simulink model "SegheriaSCADA2"  (R2024b)
settings: Solver=FixedStepAuto  StartTime=0.0  StopTime=2000  FixedStep=0.025  RelTol=1e-3
values from neighbouring files (symbols this model uses):
  b = t + 2*s    (= 3.6)    [ParametriSegheria.m]    (also in ParametriSegheriaDinamica.m; main_param_CLASSIC.m; main_param_SCADA.m)
  b2 = t2 + 2*s2    (= 10)    [ParametriSegheria.m]    (also in ParametriSegheriaDinamica.m; main_param_CLASSIC.m; main_param_SCADA.m)
  h_index = [70, 80, 90, 100]    [ParametriSegheria.m]    (also in ParametriSegheriaDinamica.m = [80, 90, 100]; main_param_CLASSIC.m = [80, 90, 100, 110]; main_param_SCADA.m = [80, 90, 100, 110])
  h_start_1 = 1    [main_param_CLASSIC.m]
  h_start_2 = 2    [main_param_CLASSIC.m]
  h_start_3 = 3    [main_param_CLASSIC.m]
  h_start_4 = 1    [main_param_CLASSIC.m]
  h_start_5 = 2    [main_param_CLASSIC.m]
  h_start_6 = 3    [main_param_CLASSIC.m]
  i_id = 60    [ParametriSegheria.m]
  i_id2 = 60    [ParametriSegheria.m]
  i_max = 100    [ParametriSegheria.m]
  kc = [0 35 40 50 55 90]    [ParametriSegheria.m]    (also in ParametriSegheriaDinamica.m = [0, 25, 30, 35, 50, 70]; main_param_CLASSIC.m = [0, 25, 30, 35, 50, 70]; main_param_SCADA.m = [0, 25, 30, 35, 50, 70])
  Kt = 2    [ParametriSegheria.m]    (also in ParametriSegheriaDinamica.m = 10000; main_param_CLASSIC.m = 10000; main_param_SCADA.m = 10000)
  Kt2 = 5    [ParametriSegheria.m]    (also in ParametriSegheriaDinamica.m = 4500; main_param_CLASSIC.m = 4500; main_param_SCADA.m = 4500)
  l_index = [20, 30, 40, 50]    [ParametriSegheria.m]    (also in ParametriSegheriaDinamica.m = [30, 40, 50]; main_param_CLASSIC.m = [30, 40, 50, 60]; main_param_SCADA.m = [30, 40, 50, 60])
  l_start_1 = 1    [main_param_CLASSIC.m]
  l_start_2 = 1    [main_param_CLASSIC.m]
  l_start_3 = 1    [main_param_CLASSIC.m]
  l_start_4 = 1    [main_param_CLASSIC.m]
  l_start_5 = 1    [main_param_CLASSIC.m]
  l_start_6 = 1    [main_param_CLASSIC.m]
  Lt = 4    [ParametriSegheria.m]    (also in ParametriSegheriaDinamica.m; main_param_CLASSIC.m; main_param_SCADA.m)
  Mag_D1 = [0 randi([220 500], 1, 40)]    [ParametriSegheria.m]    (also in ParametriSegheriaDinamica.m = [0 randi([200 500], 1, N_log)]; main_param_CLASSIC.m = [0 randi([200 500], 1, N_log)]; main_param_SCADA.m = [0 randi([200 500], 1, N_log)])
  Mag_D2 = [0 randi([220 500], 1, 40)]    [ParametriSegheria.m]    (also in ParametriSegheriaDinamica.m = [0 randi([200 500], 1, N_log)]; main_param_CLASSIC.m = [0 randi([200 500], 1, N_log)]; main_param_SCADA.m = [0 randi([200 500], 1, N_log)])
  Mag_D3 = [0 randi([220 500], 1, 40)]    [ParametriSegheria.m]    (also in ParametriSegheriaDinamica.m = [0 randi([200 500], 1, N_log)]; main_param_CLASSIC.m = [0 randi([200 500], 1, N_log)]; main_param_SCADA.m = [0 randi([200 500], 1, N_log)])
  Mag_legno1 = [0 randi([1 5], 1, 40)]    [ParametriSegheria.m]    (also in ParametriSegheriaDinamica.m = [0 randi([1 5], 1, N_log)]; main_param_CLASSIC.m = [0 randi([1 5], 1, N_log)]; main_param_SCADA.m = [0 randi([1 5], 1, N_log)])
  Mag_legno2 = [0 randi([1 5], 1, 40)]    [ParametriSegheria.m]    (also in ParametriSegheriaDinamica.m = [0 randi([1 5], 1, N_log)]; main_param_CLASSIC.m = [0 randi([1 5], 1, N_log)]; main_param_SCADA.m = [0 randi([1 5], 1, N_log)])
  Mag_legno3 = [0 randi([1 5], 1, 40)]    [ParametriSegheria.m]    (also in ParametriSegheriaDinamica.m = [0 randi([1 5], 1, N_log)]; main_param_CLASSIC.m = [0 randi([1 5], 1, N_log)]; main_param_SCADA.m = [0 randi([1 5], 1, N_log)])
  n_sottili = 4    [ParametriSegheria.m]
  omega = 50    [ParametriSegheria.m]
  omega2 = 3000*(2*pi/60)    (= 314.159265359)    [ParametriSegheria.m]
  SR = Rs/Rm    (= 5.33333333333)    [ParametriSegheria.m]    (also in ParametriSegheriaDinamica.m; main_param_CLASSIC.m; main_param_SCADA.m)
  SR2 = Rc/Rm2    (= 4)    [ParametriSegheria.m]    (also in ParametriSegheriaDinamica.m; main_param_CLASSIC.m; main_param_SCADA.m)
  thrsh = 40    [ParametriSegheria.m]
  Tloss = Tatt+ Tdamp    (= 17.3333333333)    [ParametriSegheria.m]
  Tloss2 = Tatt2+ Tdamp2    (= 66.8318530718)    [ParametriSegheria.m]
libraries: simulink x15, slpidlib x9
(part 2 of 3)

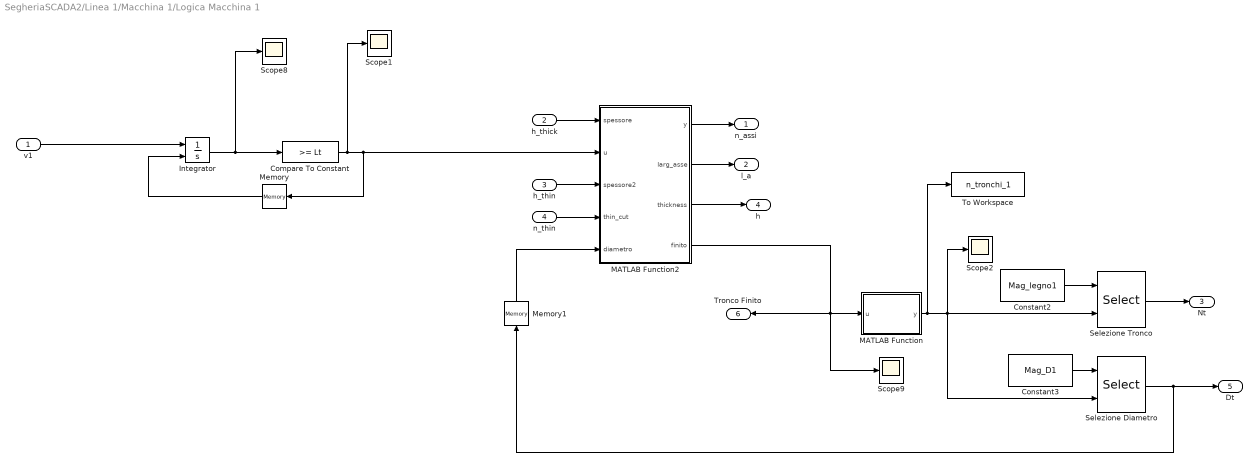
== system SegheriaSCADA2/Linea 1/Macchina 1/Logica Macchina 1 ==
  v1 : Inport
  h_thick : Inport  Port=2
  h_thin : Inport  Port=3
  n_thin : Inport  Port=4
  Compare To Constant : simulink/Logic and Bit Operations/Compare To Constant  relop=>=  const=Lt  OutDataTypeStr=boolean
  Constant2 : Constant  Value=Mag_legno1
  Constant3 : Constant  Value=Mag_D1
  Integrator : Integrator  ExternalReset=rising
  MATLAB Function : MATLAB Function  TreatAsAtomicUnit=on
  MATLAB Function2 : MATLAB Function  TreatAsAtomicUnit=on
  Memory : Memory
  Memory1 : Memory
  Scope{1..2,8..9} (4 alike) : Scope
  Selezione Diametro : Selector  IndexMode=Zero-based  InputPortWidth=length(Mag_D1)  IndexOptions=Index vector (port)  Indices=[1 3]  OutputSizes=1
  Selezione Tronco : Selector  IndexMode=Zero-based  InputPortWidth=length(Mag_legno1)  IndexOptions=Index vector (port)  Indices=[1 3]  OutputSizes=1
  To Workspace : ToWorkspace  VariableName=n_tronchi_1  SaveFormat=Timeseries  SampleTime=-1
  n_assi : Outport
  l_a : Outport  Port=2
  Nt : Outport  Port=3
  h : Outport  Port=4
  Dt : Outport  Port=5
  Tronco Finito : Outport  Port=6
  wires:
  Selezione Diametro/1 -> Dt/1, Memory1/1
  MATLAB Function2/4(finito) -> Scope9/1, Tronco Finito/1, MATLAB Function/1(u)
  Memory/1 -> Integrator/2
  Memory1/1 -> MATLAB Function2/5(diametro)
  Constant2/1 -> Selezione Tronco/1
  v1/1 -> Integrator/1
  Integrator/1 -> Compare To Constant/1, Scope8/1
  Constant3/1 -> Selezione Diametro/1
  MATLAB Function/1(y) -> To Workspace/1, Selezione Diametro/2, Scope2/1, Selezione Tronco/2
  MATLAB Function2/1(y) -> n_assi/1
  Selezione Tronco/1 -> Nt/1
  MATLAB Function2/2(larg_asse) -> l_a/1
  Compare To Constant/1 -> Scope1/1, Memory/1, MATLAB Function2/2(u)
  h_thick/1 -> MATLAB Function2/1(spessore)
  h_thin/1 -> MATLAB Function2/3(spessore2)
  n_thin/1 -> MATLAB Function2/4(thin_cut)
  MATLAB Function2/3(thickness) -> h/1

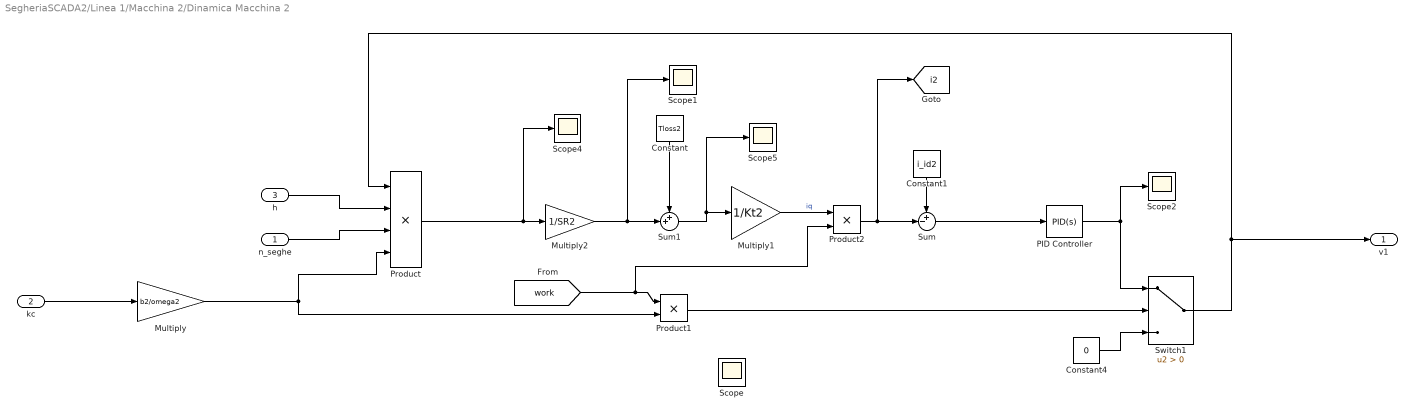
== system SegheriaSCADA2/Linea 1/Macchina 2/Dinamica Macchina 2 ==
  n_seghe : Inport
  kc : Inport  Port=2
  h : Inport  Port=3
  Constant : Constant  Value=Tloss2
  Constant1 : Constant  Value=i_id2
  Constant4 : Constant  Value=0
  Multiply : Gain  Gain=b2/omega2
  Multiply1 : Gain  Gain=1/Kt2
  Multiply2 : Gain  Gain=1/SR2
  PID Controller : slpidlib/PID Controller  Controller=PID  Form=Parallel  TimeDomain=Continuous-time  UseExternalTs=off  SampleTime=-1  IntegratorMethod=Forward Euler  FilterMethod=Forward Euler  ControllerParametersSource=internal  P=0.1  I=0  UseKiTs=off  D=0  UseExternalDerivativeSource=off  N=100  UseFilter=on  TunerSelectOption=Transfer Function Based (PID Tuner App)  InitialConditionSource=internal  InitialConditionForIntegrator=0  InitialConditionForFilter=0  DifferentiatorICPrevScaledInput=0  ExternalReset=none  TrackingMode=off  Kt=1  LimitOutput=off  SatLimitsSource=internal  UpperSaturationLimit=1.7  LowerSaturationLimit=0  LinearizeAsGain=on  AntiWindupMode=none  Kb=1  LimitIntegrator=off  UpperIntegratorSaturationLimit=inf  LowerIntegratorSaturationLimit=-inf  POutMin=[]  POutMax=[]  IOutMin=[]  IOutMax=[]  DOutMin=[]  DOutMax=[]  NOutMin=[]  NOutMax=[]  SumOutMin=[]  SumOutMax=[]  SaturationOutMin=[]  SaturationOutMax=[]  PParamMin=[]  PParamMax=[]  IParamMin=[]  IParamMax=[]  DParamMin=[]  DParamMax=[]  NParamMin=[]  NParamMax=[]  KbParamMin=[]  KbParamMax=[]  KtParamMin=[]  KtParamMax=[]  KbOutMin=[]  KbOutMax=[]  KtOutMin=[]  KtOutMax=[]  IntegratorOutMin=[]  IntegratorOutMax=[]  FilterOutMin=[]  FilterOutMax=[]  SumI1OutMin=[]  SumI1OutMax=[]  SumI2OutMin=[]  SumI2OutMax=[]  SumI3OutMin=[]  SumI3OutMax=[]  SumI4OutMin=[]  SumI4OutMax=[]  SumDOutMin=[]  SumDOutMax=[]  DifferentiatorOutMin=[]  DifferentiatorOutMax=[]  FilterDiffOutCoefMin=[]  FilterDiffOutCoefMax=[]  ReciprocalOutMin=[]  ReciprocalOutMax=[]  SumDenOutMin=[]  SumDenOutMax=[]  SumNumOutMin=[]  SumNumOutMax=[]  DivideOutMin=[]  DivideOutMax=[]  UdiffTsProdOutMin=[]  UdiffTsProdOutMax=[]  NTsProdOutMin=[]  NTsProdOutMax=[]  UintegralTsProdOutMin=[]  UintegralTsProdOutMax=[]  UngainTsProdOutMin=[]  UngainTsProdOutMax=[]  ClampingZeroOutDataTypeStr=Inherit: Inherit via back propagation  ClampingZeroOutMin=[]  ClampingZeroOutMax=[]  FilterDenConstantOutDataTypeStr=Inherit: Inherit via back propagation  FilterDenConstantOutMin=[]  FilterDenConstantOutMax=[]  PCopyOutDataTypeStr=Inherit: Inherit via back propagation  PCopyOutMin=[]  PCopyOutMax=[]  NCopyOutDataTypeStr=Inherit: Inherit via back propagation  NCopyOutMin=[]  NCopyOutMax=[]  IntegratorContinuousStateAttributes=''  IntegratorStateMustResolveToSignalObject=off  IntegratorRTWStateStorageClass=Auto  FilterContinuousStateAttributes=''  FilterStateMustResolveToSignalObject=off  FilterRTWStateStorageClass=Auto  ParallelPVariant=InternalParameters  IdealPVariant=Disabled  IVariant=InternalParameters  DVariant=InternalParameters  IntegratorVariant=Continuous  SatVariant=Disabled  AWVariant=Passthrough  PCopyVariant=Disabled  TRVariant=Disabled  FdbkBlocksVariant=Forward  IdealPFdbkVariant=Disabled  SatFdbkVariant=Disabled  DerivativeFilterVariant=ContFilter  NVariant=InternalParameters  NCopyVariant=Disabled  FilterICVariant=InternalICsFilter  IntegratorICVariant=InternalICs  ExternalResetVariant=Disabled  TRSumVariant=Passthrough  SumFdbkVariant=Disabled  SumVariant=Sum_PID  TsampFilterVariant=InternalTs  TsampNgainVariant=Passthrough  TsampIntegralVariant=Disabled_SignalSpec  ExternalSaturationOutDataTypeStr=Inherit: Same as second input  DerivativeSourceVariant=ErrorSignal  PreIntVariant=InternalPreInt
  Product : Product  Inputs=4
  Product1 : Product
  Product2 : Product
  Scope{,1..2,4..5} (5 alike) : Scope
  Sum : Sum  Inputs=+-|
  Sum1 : Sum  Inputs=++|
  Switch1 : Switch  Criteria=u2 > Threshold  SaturateOnIntegerOverflow=off  InputSameDT=off
  v1 : Outport
  tag scope: i2=global
  wires:
  Constant4/1 -> Switch1/3
  Product/1 -> Scope4/1, Multiply2/1
  PID Controller/1 -> Switch1/1, Scope2/1
  Multiply1/1 -> Product2/1  "iq"
  kc/1 -> Multiply/1
  Switch1/1 -> v1/1, Product/1
  Constant1/1 -> Sum/1
  Sum/1 -> PID Controller/1
  Multiply2/1 -> Scope1/1, Sum1/2
  Sum1/1 -> Scope5/1, Multiply1/1
  Constant/1 -> Sum1/1
  h/1 -> Product/2
  n_seghe/1 -> Product/3
  Multiply/1 -> Product1/2, Product/4
  Product1/1 -> Switch1/2
  [work] -> Product2/2, Product1/1
  Product2/1 -> [i2], Sum/2

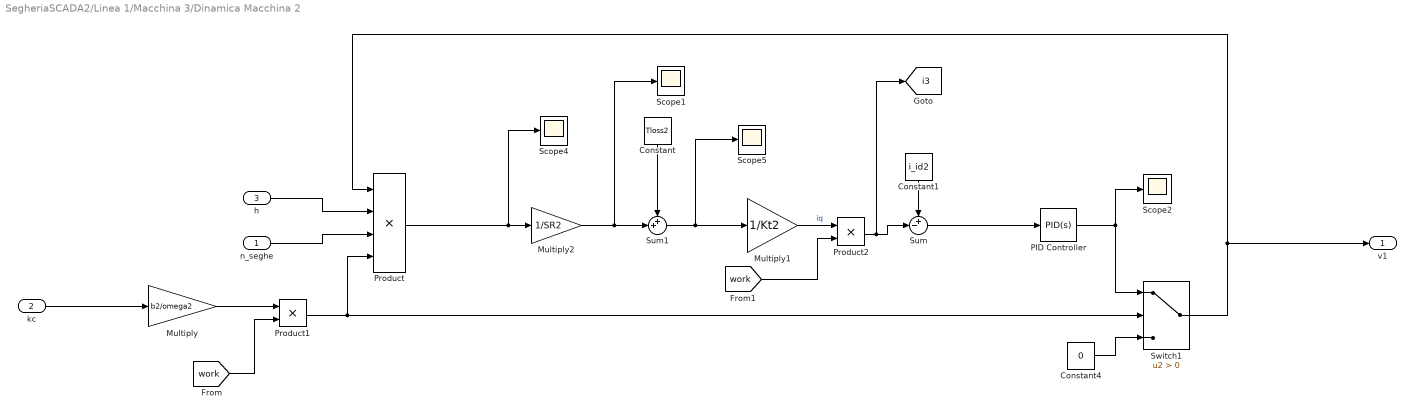
== system SegheriaSCADA2/Linea 1/Macchina 3/Dinamica Macchina 2 ==
  n_seghe : Inport
  kc : Inport  Port=2
  h : Inport  Port=3
  Constant : Constant  Value=Tloss2
  Constant1 : Constant  Value=i_id2
  Constant4 : Constant  Value=0
  Multiply : Gain  Gain=b2/omega2
  Multiply1 : Gain  Gain=1/Kt2
  Multiply2 : Gain  Gain=1/SR2
  PID Controller : slpidlib/PID Controller  Controller=PID  Form=Parallel  TimeDomain=Continuous-time  UseExternalTs=off  SampleTime=-1  IntegratorMethod=Forward Euler  FilterMethod=Forward Euler  ControllerParametersSource=internal  P=0.1  I=0  UseKiTs=off  D=0  UseExternalDerivativeSource=off  N=100  UseFilter=on  TunerSelectOption=Transfer Function Based (PID Tuner App)  InitialConditionSource=internal  InitialConditionForIntegrator=0  InitialConditionForFilter=0  DifferentiatorICPrevScaledInput=0  ExternalReset=none  TrackingMode=off  Kt=1  LimitOutput=off  SatLimitsSource=internal  UpperSaturationLimit=1.7  LowerSaturationLimit=0  LinearizeAsGain=on  AntiWindupMode=none  Kb=1  LimitIntegrator=off  UpperIntegratorSaturationLimit=inf  LowerIntegratorSaturationLimit=-inf  POutMin=[]  POutMax=[]  IOutMin=[]  IOutMax=[]  DOutMin=[]  DOutMax=[]  NOutMin=[]  NOutMax=[]  SumOutMin=[]  SumOutMax=[]  SaturationOutMin=[]  SaturationOutMax=[]  PParamMin=[]  PParamMax=[]  IParamMin=[]  IParamMax=[]  DParamMin=[]  DParamMax=[]  NParamMin=[]  NParamMax=[]  KbParamMin=[]  KbParamMax=[]  KtParamMin=[]  KtParamMax=[]  KbOutMin=[]  KbOutMax=[]  KtOutMin=[]  KtOutMax=[]  IntegratorOutMin=[]  IntegratorOutMax=[]  FilterOutMin=[]  FilterOutMax=[]  SumI1OutMin=[]  SumI1OutMax=[]  SumI2OutMin=[]  SumI2OutMax=[]  SumI3OutMin=[]  SumI3OutMax=[]  SumI4OutMin=[]  SumI4OutMax=[]  SumDOutMin=[]  SumDOutMax=[]  DifferentiatorOutMin=[]  DifferentiatorOutMax=[]  FilterDiffOutCoefMin=[]  FilterDiffOutCoefMax=[]  ReciprocalOutMin=[]  ReciprocalOutMax=[]  SumDenOutMin=[]  SumDenOutMax=[]  SumNumOutMin=[]  SumNumOutMax=[]  DivideOutMin=[]  DivideOutMax=[]  UdiffTsProdOutMin=[]  UdiffTsProdOutMax=[]  NTsProdOutMin=[]  NTsProdOutMax=[]  UintegralTsProdOutMin=[]  UintegralTsProdOutMax=[]  UngainTsProdOutMin=[]  UngainTsProdOutMax=[]  ClampingZeroOutDataTypeStr=Inherit: Inherit via back propagation  ClampingZeroOutMin=[]  ClampingZeroOutMax=[]  FilterDenConstantOutDataTypeStr=Inherit: Inherit via back propagation  FilterDenConstantOutMin=[]  FilterDenConstantOutMax=[]  PCopyOutDataTypeStr=Inherit: Inherit via back propagation  PCopyOutMin=[]  PCopyOutMax=[]  NCopyOutDataTypeStr=Inherit: Inherit via back propagation  NCopyOutMin=[]  NCopyOutMax=[]  IntegratorContinuousStateAttributes=''  IntegratorStateMustResolveToSignalObject=off  IntegratorRTWStateStorageClass=Auto  FilterContinuousStateAttributes=''  FilterStateMustResolveToSignalObject=off  FilterRTWStateStorageClass=Auto  ParallelPVariant=InternalParameters  IdealPVariant=Disabled  IVariant=InternalParameters  DVariant=InternalParameters  IntegratorVariant=Continuous  SatVariant=Disabled  AWVariant=Passthrough  PCopyVariant=Disabled  TRVariant=Disabled  FdbkBlocksVariant=Forward  IdealPFdbkVariant=Disabled  SatFdbkVariant=Disabled  DerivativeFilterVariant=ContFilter  NVariant=InternalParameters  NCopyVariant=Disabled  FilterICVariant=InternalICsFilter  IntegratorICVariant=InternalICs  ExternalResetVariant=Disabled  TRSumVariant=Passthrough  SumFdbkVariant=Disabled  SumVariant=Sum_PID  TsampFilterVariant=InternalTs  TsampNgainVariant=Passthrough  TsampIntegralVariant=Disabled_SignalSpec  ExternalSaturationOutDataTypeStr=Inherit: Same as second input  DerivativeSourceVariant=ErrorSignal  PreIntVariant=InternalPreInt
  Product : Product  Inputs=4
  Product1 : Product
  Product2 : Product
  Scope{1..2,4..5} (4 alike) : Scope
  Sum : Sum  Inputs=+-|
  Sum1 : Sum  Inputs=++|
  Switch1 : Switch  Criteria=u2 > Threshold  SaturateOnIntegerOverflow=off  InputSameDT=off
  v1 : Outport
  tag scope: i3=global
  wires:
  n_seghe/1 -> Product/3
  h/1 -> Product/2
  Constant/1 -> Sum1/1
  Sum1/1 -> Multiply1/1, Scope5/1
  Multiply2/1 -> Sum1/2, Scope1/1
  Sum/1 -> PID Controller/1
  Constant1/1 -> Sum/1
  Switch1/1 -> Product/1, v1/1
  kc/1 -> Multiply/1
  Multiply1/1 -> Product2/1  "iq"
  PID Controller/1 -> Scope2/1, Switch1/1
  Product/1 -> Multiply2/1, Scope4/1
  Constant4/1 -> Switch1/3
  Multiply/1 -> Product1/1
  Product1/1 -> Switch1/2, Product/4
  [work] -> Product1/2
  Product2/1 -> [i3], Sum/2
  [work] -> Product2/2

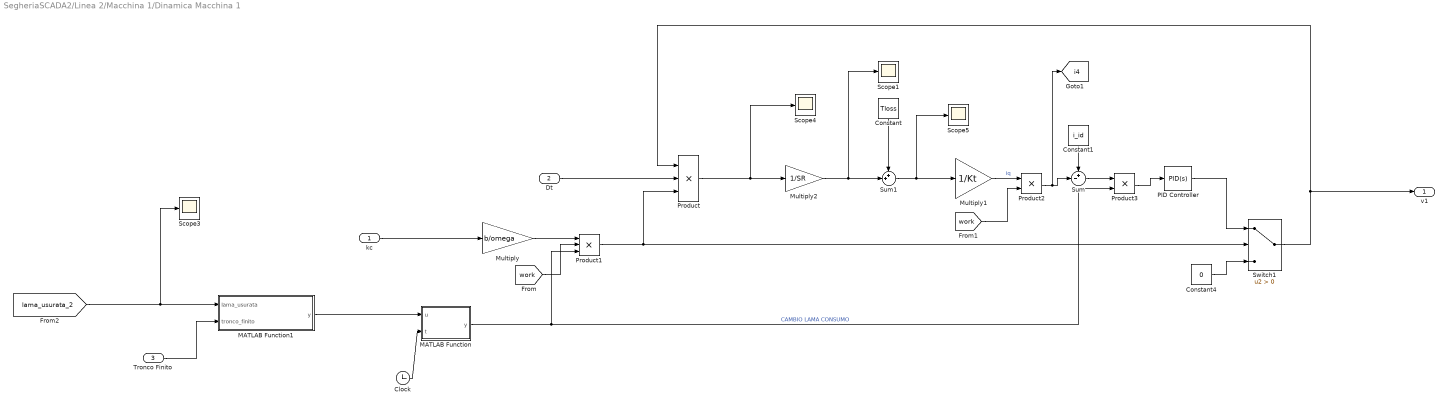
== system SegheriaSCADA2/Linea 2/Macchina 1/Dinamica Macchina 1 ==
  kc : Inport
  Dt : Inport  Port=2
  Tronco Finito : Inport  Port=3
  Clock : Clock
  Constant : Constant  Value=Tloss
  Constant1 : Constant  Value=i_id
  Constant4 : Constant  Value=0
  MATLAB Function : MATLAB Function  TreatAsAtomicUnit=on
  MATLAB Function1 : MATLAB Function  TreatAsAtomicUnit=on
  Multiply : Gain  Gain=b/omega
  Multiply1 : Gain  Gain=1/Kt
  Multiply2 : Gain  Gain=1/SR
  PID Controller : slpidlib/PID Controller  Controller=PID  Form=Parallel  TimeDomain=Continuous-time  UseExternalTs=off  SampleTime=-1  IntegratorMethod=Forward Euler  FilterMethod=Forward Euler  ControllerParametersSource=internal  P=0  I=0.0048685791703887  UseKiTs=off  D=0  UseExternalDerivativeSource=off  N=100  UseFilter=on  TunerSelectOption=Transfer Function Based (PID Tuner App)  InitialConditionSource=internal  InitialConditionForIntegrator=0  InitialConditionForFilter=0  DifferentiatorICPrevScaledInput=0  ExternalReset=none  TrackingMode=off  Kt=1  LimitOutput=on  SatLimitsSource=internal  UpperSaturationLimit=i_max  LowerSaturationLimit=-inf  LinearizeAsGain=on  AntiWindupMode=none  Kb=1  LimitIntegrator=off  UpperIntegratorSaturationLimit=inf  LowerIntegratorSaturationLimit=-inf  POutMin=[]  POutMax=[]  IOutMin=[]  IOutMax=[]  DOutMin=[]  DOutMax=[]  NOutMin=[]  NOutMax=[]  SumOutMin=[]  SumOutMax=[]  SaturationOutMin=[]  SaturationOutMax=[]  PParamMin=[]  PParamMax=[]  IParamMin=[]  IParamMax=[]  DParamMin=[]  DParamMax=[]  NParamMin=[]  NParamMax=[]  KbParamMin=[]  KbParamMax=[]  KtParamMin=[]  KtParamMax=[]  KbOutMin=[]  KbOutMax=[]  KtOutMin=[]  KtOutMax=[]  IntegratorOutMin=[]  IntegratorOutMax=[]  FilterOutMin=[]  FilterOutMax=[]  SumI1OutMin=[]  SumI1OutMax=[]  SumI2OutMin=[]  SumI2OutMax=[]  SumI3OutMin=[]  SumI3OutMax=[]  SumI4OutMin=[]  SumI4OutMax=[]  SumDOutMin=[]  SumDOutMax=[]  DifferentiatorOutMin=[]  DifferentiatorOutMax=[]  FilterDiffOutCoefMin=[]  FilterDiffOutCoefMax=[]  ReciprocalOutMin=[]  ReciprocalOutMax=[]  SumDenOutMin=[]  SumDenOutMax=[]  SumNumOutMin=[]  SumNumOutMax=[]  DivideOutMin=[]  DivideOutMax=[]  UdiffTsProdOutMin=[]  UdiffTsProdOutMax=[]  NTsProdOutMin=[]  NTsProdOutMax=[]  UintegralTsProdOutMin=[]  UintegralTsProdOutMax=[]  UngainTsProdOutMin=[]  UngainTsProdOutMax=[]  ClampingZeroOutDataTypeStr=Inherit: Inherit via back propagation  ClampingZeroOutMin=[]  ClampingZeroOutMax=[]  FilterDenConstantOutDataTypeStr=Inherit: Inherit via back propagation  FilterDenConstantOutMin=[]  FilterDenConstantOutMax=[]  PCopyOutDataTypeStr=Inherit: Inherit via back propagation  PCopyOutMin=[]  PCopyOutMax=[]  NCopyOutDataTypeStr=Inherit: Inherit via back propagation  NCopyOutMin=[]  NCopyOutMax=[]  IntegratorContinuousStateAttributes=''  IntegratorStateMustResolveToSignalObject=off  IntegratorRTWStateStorageClass=Auto  FilterContinuousStateAttributes=''  FilterStateMustResolveToSignalObject=off  FilterRTWStateStorageClass=Auto  ParallelPVariant=InternalParameters  IdealPVariant=Disabled  IVariant=InternalParameters  DVariant=InternalParameters  IntegratorVariant=Continuous  SatVariant=Enabled  AWVariant=Passthrough  PCopyVariant=Disabled  TRVariant=Disabled  FdbkBlocksVariant=Forward  IdealPFdbkVariant=Disabled  SatFdbkVariant=Disabled  DerivativeFilterVariant=ContFilter  NVariant=InternalParameters  NCopyVariant=Disabled  FilterICVariant=InternalICsFilter  IntegratorICVariant=InternalICs  ExternalResetVariant=Disabled  TRSumVariant=Passthrough  SumFdbkVariant=Disabled  SumVariant=Sum_PID  TsampFilterVariant=InternalTs  TsampNgainVariant=Passthrough  TsampIntegralVariant=Disabled_SignalSpec  ExternalSaturationOutDataTypeStr=Inherit: Same as second input  DerivativeSourceVariant=ErrorSignal  PreIntVariant=InternalPreInt
  Product : Product  Inputs=3
  Product1 : Product  Inputs=3
  Product2 : Product
  Product3 : Product
  Scope{1,3..5} (4 alike) : Scope
  Sum : Sum  Inputs=+-|
  Sum1 : Sum  Inputs=++|
  Switch1 : Switch  Criteria=u2 > Threshold  SaturateOnIntegerOverflow=off  InputSameDT=off
  v1 : Outport
  tag scope: i4=global
  wires:
  Constant4/1 -> Switch1/3
  Product/1 -> Scope4/1, Multiply2/1
  PID Controller/1 -> Switch1/1
  Multiply1/1 -> Product2/1  "iq"
  kc/1 -> Multiply/1
  Switch1/1 -> v1/1, Product/1
  Constant1/1 -> Sum/1
  Multiply2/1 -> Sum1/2, Scope1/1
  Sum1/1 -> Scope5/1, Multiply1/1
  Constant/1 -> Sum1/1
  Dt/1 -> Product/2
  Multiply/1 -> Product1/1
  Product1/1 -> Switch1/2, Product/3
  [work] -> Product1/2
  MATLAB Function/1(y) -> Product3/2, Product1/3  "CAMBIO LAMA CONSUMO"
  Clock/1 -> MATLAB Function/2(t)
  Tronco Finito/1 -> MATLAB Function1/2(tronco_finito)
  [lama_usurata_2] -> Scope3/1, MATLAB Function1/1(lama_usurata)
  MATLAB Function1/1(y) -> MATLAB Function/1(u)
  Product2/1 -> [i4], Sum/2
  [work] -> Product2/2
  Sum/1 -> Product3/1
  Product3/1 -> PID Controller/1

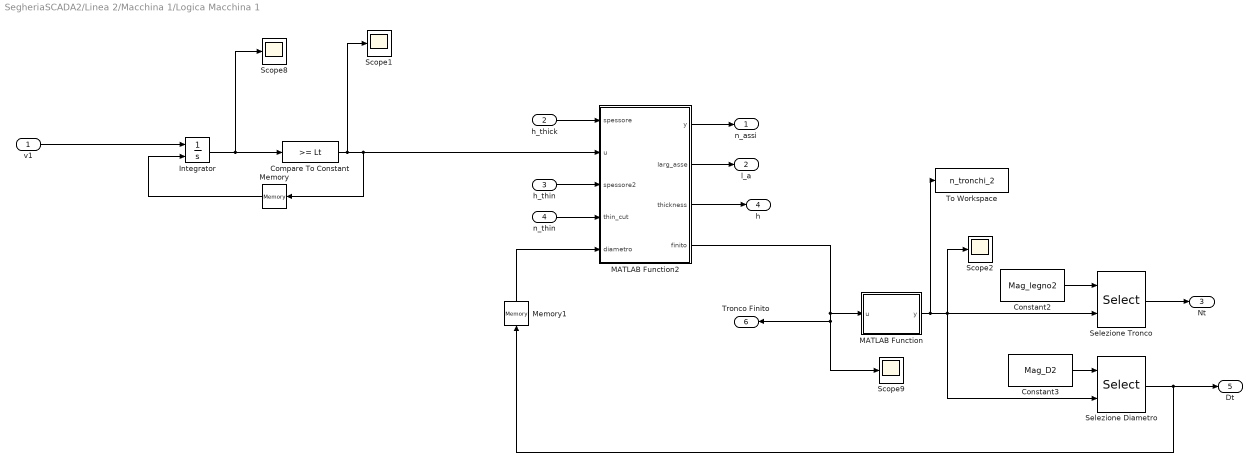
== system SegheriaSCADA2/Linea 2/Macchina 1/Logica Macchina 1 ==
  v1 : Inport
  h_thick : Inport  Port=2
  h_thin : Inport  Port=3
  n_thin : Inport  Port=4
  Compare To Constant : simulink/Logic and Bit Operations/Compare To Constant  relop=>=  const=Lt  OutDataTypeStr=boolean
  Constant2 : Constant  Value=Mag_legno2
  Constant3 : Constant  Value=Mag_D2
  Integrator : Integrator  ExternalReset=rising
  MATLAB Function : MATLAB Function  TreatAsAtomicUnit=on
  MATLAB Function2 : MATLAB Function  TreatAsAtomicUnit=on
  Memory : Memory
  Memory1 : Memory
  Scope{1..2,8..9} (4 alike) : Scope
  Selezione Diametro : Selector  IndexMode=Zero-based  InputPortWidth=length(Mag_D2)  IndexOptions=Index vector (port)  Indices=[1 3]  OutputSizes=1
  Selezione Tronco : Selector  IndexMode=Zero-based  InputPortWidth=length(Mag_legno2)  IndexOptions=Index vector (port)  Indices=[1 3]  OutputSizes=1
  To Workspace : ToWorkspace  VariableName=n_tronchi_2  SaveFormat=Timeseries  SampleTime=-1
  n_assi : Outport
  l_a : Outport  Port=2
  Nt : Outport  Port=3
  h : Outport  Port=4
  Dt : Outport  Port=5
  Tronco Finito : Outport  Port=6
  wires:
  Selezione Diametro/1 -> Dt/1, Memory1/1
  MATLAB Function2/4(finito) -> Scope9/1, Tronco Finito/1, MATLAB Function/1(u)
  Memory/1 -> Integrator/2
  Memory1/1 -> MATLAB Function2/5(diametro)
  Constant2/1 -> Selezione Tronco/1
  v1/1 -> Integrator/1
  Integrator/1 -> Compare To Constant/1, Scope8/1
  Constant3/1 -> Selezione Diametro/1
  MATLAB Function/1(y) -> To Workspace/1, Selezione Tronco/2, Selezione Diametro/2, Scope2/1
  MATLAB Function2/1(y) -> n_assi/1
  Selezione Tronco/1 -> Nt/1
  MATLAB Function2/2(larg_asse) -> l_a/1
  Compare To Constant/1 -> Scope1/1, Memory/1, MATLAB Function2/2(u)
  h_thick/1 -> MATLAB Function2/1(spessore)
  h_thin/1 -> MATLAB Function2/3(spessore2)
  n_thin/1 -> MATLAB Function2/4(thin_cut)
  MATLAB Function2/3(thickness) -> h/1

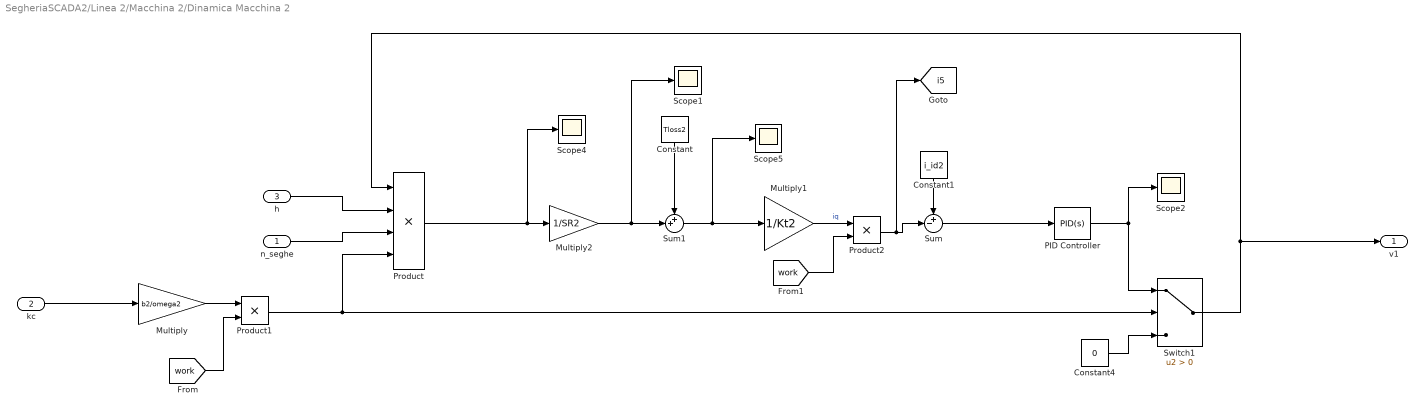
== system SegheriaSCADA2/Linea 2/Macchina 2/Dinamica Macchina 2 ==
  n_seghe : Inport
  kc : Inport  Port=2
  h : Inport  Port=3
  Constant : Constant  Value=Tloss2
  Constant1 : Constant  Value=i_id2
  Constant4 : Constant  Value=0
  Multiply : Gain  Gain=b2/omega2
  Multiply1 : Gain  Gain=1/Kt2
  Multiply2 : Gain  Gain=1/SR2
  PID Controller : slpidlib/PID Controller  Controller=PID  Form=Parallel  TimeDomain=Continuous-time  UseExternalTs=off  SampleTime=-1  IntegratorMethod=Forward Euler  FilterMethod=Forward Euler  ControllerParametersSource=internal  P=0.1  I=0  UseKiTs=off  D=0  UseExternalDerivativeSource=off  N=100  UseFilter=on  TunerSelectOption=Transfer Function Based (PID Tuner App)  InitialConditionSource=internal  InitialConditionForIntegrator=0  InitialConditionForFilter=0  DifferentiatorICPrevScaledInput=0  ExternalReset=none  TrackingMode=off  Kt=1  LimitOutput=off  SatLimitsSource=internal  UpperSaturationLimit=1.7  LowerSaturationLimit=0  LinearizeAsGain=on  AntiWindupMode=none  Kb=1  LimitIntegrator=off  UpperIntegratorSaturationLimit=inf  LowerIntegratorSaturationLimit=-inf  POutMin=[]  POutMax=[]  IOutMin=[]  IOutMax=[]  DOutMin=[]  DOutMax=[]  NOutMin=[]  NOutMax=[]  SumOutMin=[]  SumOutMax=[]  SaturationOutMin=[]  SaturationOutMax=[]  PParamMin=[]  PParamMax=[]  IParamMin=[]  IParamMax=[]  DParamMin=[]  DParamMax=[]  NParamMin=[]  NParamMax=[]  KbParamMin=[]  KbParamMax=[]  KtParamMin=[]  KtParamMax=[]  KbOutMin=[]  KbOutMax=[]  KtOutMin=[]  KtOutMax=[]  IntegratorOutMin=[]  IntegratorOutMax=[]  FilterOutMin=[]  FilterOutMax=[]  SumI1OutMin=[]  SumI1OutMax=[]  SumI2OutMin=[]  SumI2OutMax=[]  SumI3OutMin=[]  SumI3OutMax=[]  SumI4OutMin=[]  SumI4OutMax=[]  SumDOutMin=[]  SumDOutMax=[]  DifferentiatorOutMin=[]  DifferentiatorOutMax=[]  FilterDiffOutCoefMin=[]  FilterDiffOutCoefMax=[]  ReciprocalOutMin=[]  ReciprocalOutMax=[]  SumDenOutMin=[]  SumDenOutMax=[]  SumNumOutMin=[]  SumNumOutMax=[]  DivideOutMin=[]  DivideOutMax=[]  UdiffTsProdOutMin=[]  UdiffTsProdOutMax=[]  NTsProdOutMin=[]  NTsProdOutMax=[]  UintegralTsProdOutMin=[]  UintegralTsProdOutMax=[]  UngainTsProdOutMin=[]  UngainTsProdOutMax=[]  ClampingZeroOutDataTypeStr=Inherit: Inherit via back propagation  ClampingZeroOutMin=[]  ClampingZeroOutMax=[]  FilterDenConstantOutDataTypeStr=Inherit: Inherit via back propagation  FilterDenConstantOutMin=[]  FilterDenConstantOutMax=[]  PCopyOutDataTypeStr=Inherit: Inherit via back propagation  PCopyOutMin=[]  PCopyOutMax=[]  NCopyOutDataTypeStr=Inherit: Inherit via back propagation  NCopyOutMin=[]  NCopyOutMax=[]  IntegratorContinuousStateAttributes=''  IntegratorStateMustResolveToSignalObject=off  IntegratorRTWStateStorageClass=Auto  FilterContinuousStateAttributes=''  FilterStateMustResolveToSignalObject=off  FilterRTWStateStorageClass=Auto  ParallelPVariant=InternalParameters  IdealPVariant=Disabled  IVariant=InternalParameters  DVariant=InternalParameters  IntegratorVariant=Continuous  SatVariant=Disabled  AWVariant=Passthrough  PCopyVariant=Disabled  TRVariant=Disabled  FdbkBlocksVariant=Forward  IdealPFdbkVariant=Disabled  SatFdbkVariant=Disabled  DerivativeFilterVariant=ContFilter  NVariant=InternalParameters  NCopyVariant=Disabled  FilterICVariant=InternalICsFilter  IntegratorICVariant=InternalICs  ExternalResetVariant=Disabled  TRSumVariant=Passthrough  SumFdbkVariant=Disabled  SumVariant=Sum_PID  TsampFilterVariant=InternalTs  TsampNgainVariant=Passthrough  TsampIntegralVariant=Disabled_SignalSpec  ExternalSaturationOutDataTypeStr=Inherit: Same as second input  DerivativeSourceVariant=ErrorSignal  PreIntVariant=InternalPreInt
  Product : Product  Inputs=4
  Product1 : Product
  Product2 : Product
  Scope{1..2,4..5} (4 alike) : Scope
  Sum : Sum  Inputs=+-|
  Sum1 : Sum  Inputs=++|
  Switch1 : Switch  Criteria=u2 > Threshold  SaturateOnIntegerOverflow=off  InputSameDT=off
  v1 : Outport
  tag scope: i5=global
  wires:
  Constant4/1 -> Switch1/3
  Product/1 -> Scope4/1, Multiply2/1
  PID Controller/1 -> Switch1/1, Scope2/1
  Multiply1/1 -> Product2/1  "iq"
  kc/1 -> Multiply/1
  Switch1/1 -> v1/1, Product/1
  Constant1/1 -> Sum/1
  Sum/1 -> PID Controller/1
  Multiply2/1 -> Scope1/1, Sum1/2
  Sum1/1 -> Scope5/1, Multiply1/1
  Constant/1 -> Sum1/1
  h/1 -> Product/2
  n_seghe/1 -> Product/3
  Multiply/1 -> Product1/1
  Product1/1 -> Switch1/2, Product/4
  [work] -> Product1/2
  Product2/1 -> [i5], Sum/2
  [work] -> Product2/2

== system SegheriaSCADA2/Linea 2/Macchina 3/Dinamica Macchina 2 ==
  n_seghe : Inport
  kc : Inport  Port=2
  h : Inport  Port=3
  Constant : Constant  Value=Tloss2
  Constant1 : Constant  Value=i_id2
  Constant4 : Constant  Value=0
  Multiply : Gain  Gain=b2/omega2
  Multiply1 : Gain  Gain=1/Kt2
  Multiply2 : Gain  Gain=1/SR2
  PID Controller : slpidlib/PID Controller  Controller=PID  Form=Parallel  TimeDomain=Continuous-time  UseExternalTs=off  SampleTime=-1  IntegratorMethod=Forward Euler  FilterMethod=Forward Euler  ControllerParametersSource=internal  P=0.1  I=0  UseKiTs=off  D=0  UseExternalDerivativeSource=off  N=100  UseFilter=on  TunerSelectOption=Transfer Function Based (PID Tuner App)  InitialConditionSource=internal  InitialConditionForIntegrator=0  InitialConditionForFilter=0  DifferentiatorICPrevScaledInput=0  ExternalReset=none  TrackingMode=off  Kt=1  LimitOutput=off  SatLimitsSource=internal  UpperSaturationLimit=1.7  LowerSaturationLimit=0  LinearizeAsGain=on  AntiWindupMode=none  Kb=1  LimitIntegrator=off  UpperIntegratorSaturationLimit=inf  LowerIntegratorSaturationLimit=-inf  POutMin=[]  POutMax=[]  IOutMin=[]  IOutMax=[]  DOutMin=[]  DOutMax=[]  NOutMin=[]  NOutMax=[]  SumOutMin=[]  SumOutMax=[]  SaturationOutMin=[]  SaturationOutMax=[]  PParamMin=[]  PParamMax=[]  IParamMin=[]  IParamMax=[]  DParamMin=[]  DParamMax=[]  NParamMin=[]  NParamMax=[]  KbParamMin=[]  KbParamMax=[]  KtParamMin=[]  KtParamMax=[]  KbOutMin=[]  KbOutMax=[]  KtOutMin=[]  KtOutMax=[]  IntegratorOutMin=[]  IntegratorOutMax=[]  FilterOutMin=[]  FilterOutMax=[]  SumI1OutMin=[]  SumI1OutMax=[]  SumI2OutMin=[]  SumI2OutMax=[]  SumI3OutMin=[]  SumI3OutMax=[]  SumI4OutMin=[]  SumI4OutMax=[]  SumDOutMin=[]  SumDOutMax=[]  DifferentiatorOutMin=[]  DifferentiatorOutMax=[]  FilterDiffOutCoefMin=[]  FilterDiffOutCoefMax=[]  ReciprocalOutMin=[]  ReciprocalOutMax=[]  SumDenOutMin=[]  SumDenOutMax=[]  SumNumOutMin=[]  SumNumOutMax=[]  DivideOutMin=[]  DivideOutMax=[]  UdiffTsProdOutMin=[]  UdiffTsProdOutMax=[]  NTsProdOutMin=[]  NTsProdOutMax=[]  UintegralTsProdOutMin=[]  UintegralTsProdOutMax=[]  UngainTsProdOutMin=[]  UngainTsProdOutMax=[]  ClampingZeroOutDataTypeStr=Inherit: Inherit via back propagation  ClampingZeroOutMin=[]  ClampingZeroOutMax=[]  FilterDenConstantOutDataTypeStr=Inherit: Inherit via back propagation  FilterDenConstantOutMin=[]  FilterDenConstantOutMax=[]  PCopyOutDataTypeStr=Inherit: Inherit via back propagation  PCopyOutMin=[]  PCopyOutMax=[]  NCopyOutDataTypeStr=Inherit: Inherit via back propagation  NCopyOutMin=[]  NCopyOutMax=[]  IntegratorContinuousStateAttributes=''  IntegratorStateMustResolveToSignalObject=off  IntegratorRTWStateStorageClass=Auto  FilterContinuousStateAttributes=''  FilterStateMustResolveToSignalObject=off  FilterRTWStateStorageClass=Auto  ParallelPVariant=InternalParameters  IdealPVariant=Disabled  IVariant=InternalParameters  DVariant=InternalParameters  IntegratorVariant=Continuous  SatVariant=Disabled  AWVariant=Passthrough  PCopyVariant=Disabled  TRVariant=Disabled  FdbkBlocksVariant=Forward  IdealPFdbkVariant=Disabled  SatFdbkVariant=Disabled  DerivativeFilterVariant=ContFilter  NVariant=InternalParameters  NCopyVariant=Disabled  FilterICVariant=InternalICsFilter  IntegratorICVariant=InternalICs  ExternalResetVariant=Disabled  TRSumVariant=Passthrough  SumFdbkVariant=Disabled  SumVariant=Sum_PID  TsampFilterVariant=InternalTs  TsampNgainVariant=Passthrough  TsampIntegralVariant=Disabled_SignalSpec  ExternalSaturationOutDataTypeStr=Inherit: Same as second input  DerivativeSourceVariant=ErrorSignal  PreIntVariant=InternalPreInt
  Product : Product  Inputs=4
  Product1 : Product
  Product2 : Product
  Scope{1..2,4..5} (4 alike) : Scope
  Sum : Sum  Inputs=+-|
  Sum1 : Sum  Inputs=++|
  Switch1 : Switch  Criteria=u2 > Threshold  SaturateOnIntegerOverflow=off  InputSameDT=off
  v1 : Outport
  tag scope: i6=global
  wires:
  n_seghe/1 -> Product/3
  h/1 -> Product/2
  Constant/1 -> Sum1/1
  Sum1/1 -> Multiply1/1, Scope5/1
  Multiply2/1 -> Sum1/2, Scope1/1
  Sum/1 -> PID Controller/1
  Constant1/1 -> Sum/1
  Switch1/1 -> Product/1, v1/1
  kc/1 -> Multiply/1
  Multiply1/1 -> Product2/1  "iq"
  PID Controller/1 -> Scope2/1, Switch1/1
  Product/1 -> Multiply2/1, Scope4/1
  Constant4/1 -> Switch1/3
  Multiply/1 -> Product1/1
  Product1/1 -> Switch1/2, Product/4
  [work] -> Product1/2
  Product2/1 -> [i6], Sum/2
  [work] -> Product2/2

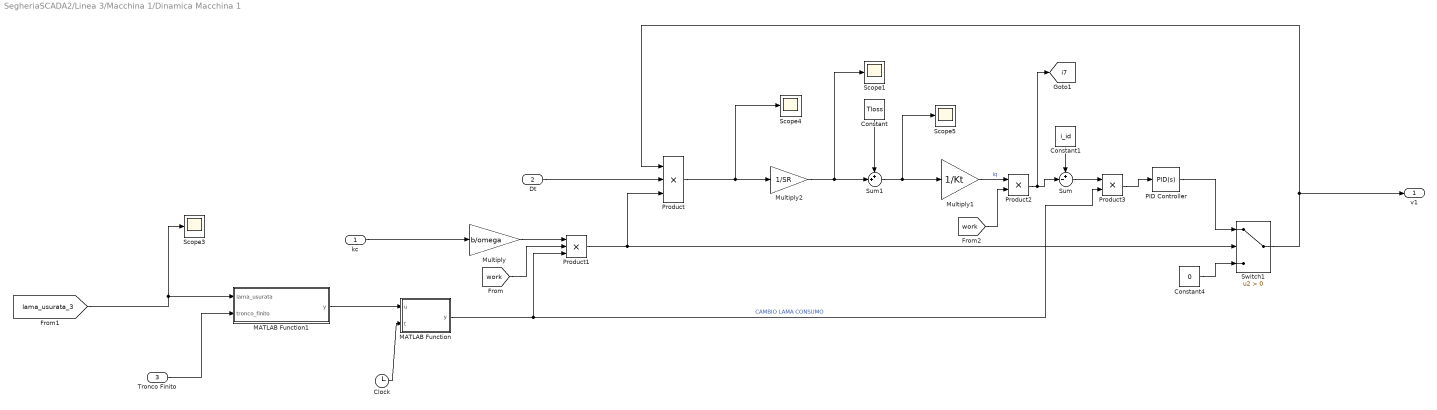
== system SegheriaSCADA2/Linea 3/Macchina 1/Dinamica Macchina 1 ==
  kc : Inport
  Dt : Inport  Port=2
  Tronco Finito : Inport  Port=3
  Clock : Clock
  Constant : Constant  Value=Tloss
  Constant1 : Constant  Value=i_id
  Constant4 : Constant  Value=0
  MATLAB Function : MATLAB Function  TreatAsAtomicUnit=on
  MATLAB Function1 : MATLAB Function  TreatAsAtomicUnit=on
  Multiply : Gain  Gain=b/omega
  Multiply1 : Gain  Gain=1/Kt
  Multiply2 : Gain  Gain=1/SR
  PID Controller : slpidlib/PID Controller  Controller=PID  Form=Parallel  TimeDomain=Continuous-time  UseExternalTs=off  SampleTime=-1  IntegratorMethod=Forward Euler  FilterMethod=Forward Euler  ControllerParametersSource=internal  P=0  I=0.0048685791703887  UseKiTs=off  D=0  UseExternalDerivativeSource=off  N=100  UseFilter=on  TunerSelectOption=Transfer Function Based (PID Tuner App)  InitialConditionSource=internal  InitialConditionForIntegrator=0  InitialConditionForFilter=0  DifferentiatorICPrevScaledInput=0  ExternalReset=none  TrackingMode=off  Kt=1  LimitOutput=on  SatLimitsSource=internal  UpperSaturationLimit=i_max  LowerSaturationLimit=-inf  LinearizeAsGain=on  AntiWindupMode=none  Kb=1  LimitIntegrator=off  UpperIntegratorSaturationLimit=inf  LowerIntegratorSaturationLimit=-inf  POutMin=[]  POutMax=[]  IOutMin=[]  IOutMax=[]  DOutMin=[]  DOutMax=[]  NOutMin=[]  NOutMax=[]  SumOutMin=[]  SumOutMax=[]  SaturationOutMin=[]  SaturationOutMax=[]  PParamMin=[]  PParamMax=[]  IParamMin=[]  IParamMax=[]  DParamMin=[]  DParamMax=[]  NParamMin=[]  NParamMax=[]  KbParamMin=[]  KbParamMax=[]  KtParamMin=[]  KtParamMax=[]  KbOutMin=[]  KbOutMax=[]  KtOutMin=[]  KtOutMax=[]  IntegratorOutMin=[]  IntegratorOutMax=[]  FilterOutMin=[]  FilterOutMax=[]  SumI1OutMin=[]  SumI1OutMax=[]  SumI2OutMin=[]  SumI2OutMax=[]  SumI3OutMin=[]  SumI3OutMax=[]  SumI4OutMin=[]  SumI4OutMax=[]  SumDOutMin=[]  SumDOutMax=[]  DifferentiatorOutMin=[]  DifferentiatorOutMax=[]  FilterDiffOutCoefMin=[]  FilterDiffOutCoefMax=[]  ReciprocalOutMin=[]  ReciprocalOutMax=[]  SumDenOutMin=[]  SumDenOutMax=[]  SumNumOutMin=[]  SumNumOutMax=[]  DivideOutMin=[]  DivideOutMax=[]  UdiffTsProdOutMin=[]  UdiffTsProdOutMax=[]  NTsProdOutMin=[]  NTsProdOutMax=[]  UintegralTsProdOutMin=[]  UintegralTsProdOutMax=[]  UngainTsProdOutMin=[]  UngainTsProdOutMax=[]  ClampingZeroOutDataTypeStr=Inherit: Inherit via back propagation  ClampingZeroOutMin=[]  ClampingZeroOutMax=[]  FilterDenConstantOutDataTypeStr=Inherit: Inherit via back propagation  FilterDenConstantOutMin=[]  FilterDenConstantOutMax=[]  PCopyOutDataTypeStr=Inherit: Inherit via back propagation  PCopyOutMin=[]  PCopyOutMax=[]  NCopyOutDataTypeStr=Inherit: Inherit via back propagation  NCopyOutMin=[]  NCopyOutMax=[]  IntegratorContinuousStateAttributes=''  IntegratorStateMustResolveToSignalObject=off  IntegratorRTWStateStorageClass=Auto  FilterContinuousStateAttributes=''  FilterStateMustResolveToSignalObject=off  FilterRTWStateStorageClass=Auto  ParallelPVariant=InternalParameters  IdealPVariant=Disabled  IVariant=InternalParameters  DVariant=InternalParameters  IntegratorVariant=Continuous  SatVariant=Enabled  AWVariant=Passthrough  PCopyVariant=Disabled  TRVariant=Disabled  FdbkBlocksVariant=Forward  IdealPFdbkVariant=Disabled  SatFdbkVariant=Disabled  DerivativeFilterVariant=ContFilter  NVariant=InternalParameters  NCopyVariant=Disabled  FilterICVariant=InternalICsFilter  IntegratorICVariant=InternalICs  ExternalResetVariant=Disabled  TRSumVariant=Passthrough  SumFdbkVariant=Disabled  SumVariant=Sum_PID  TsampFilterVariant=InternalTs  TsampNgainVariant=Passthrough  TsampIntegralVariant=Disabled_SignalSpec  ExternalSaturationOutDataTypeStr=Inherit: Same as second input  DerivativeSourceVariant=ErrorSignal  PreIntVariant=InternalPreInt
  Product : Product  Inputs=3
  Product1 : Product  Inputs=3
  Product2 : Product
  Product3 : Product
  Scope{1,3..5} (4 alike) : Scope
  Sum : Sum  Inputs=+-|
  Sum1 : Sum  Inputs=++|
  Switch1 : Switch  Criteria=u2 > Threshold  SaturateOnIntegerOverflow=off  InputSameDT=off
  v1 : Outport
  tag scope: i7=global
  wires:
  [work] -> Product1/2
  Product1/1 -> Product/3, Switch1/2
  Multiply/1 -> Product1/1
  Dt/1 -> Product/2
  Constant/1 -> Sum1/1
  Sum1/1 -> Multiply1/1, Scope5/1
  Multiply2/1 -> Scope1/1, Sum1/2
  Constant1/1 -> Sum/1
  Switch1/1 -> Product/1, v1/1
  kc/1 -> Multiply/1
  Multiply1/1 -> Product2/1  "iq"
  PID Controller/1 -> Switch1/1
  Product/1 -> Multiply2/1, Scope4/1
  Constant4/1 -> Switch1/3
  Clock/1 -> MATLAB Function/2(t)
  Tronco Finito/1 -> MATLAB Function1/2(tronco_finito)
  [lama_usurata_3] -> MATLAB Function1/1(lama_usurata), Scope3/1
  MATLAB Function1/1(y) -> MATLAB Function/1(u)
  Product2/1 -> [i7], Sum/2
  [work] -> Product2/2
  Sum/1 -> Product3/1
  Product3/1 -> PID Controller/1
  MATLAB Function/1(y) -> Product3/2, Product1/3  "CAMBIO LAMA CONSUMO"

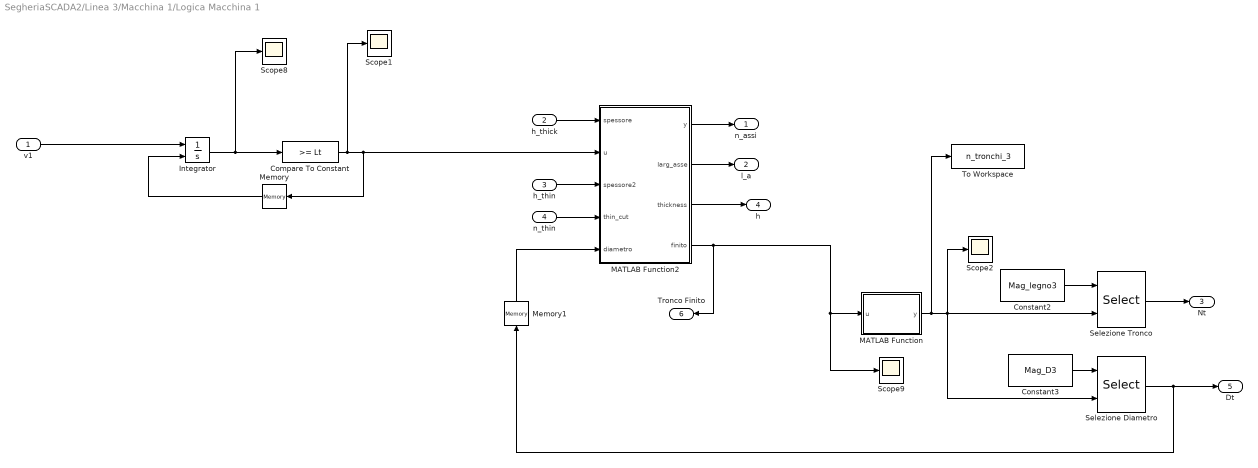
== system SegheriaSCADA2/Linea 3/Macchina 1/Logica Macchina 1 ==
  v1 : Inport
  h_thick : Inport  Port=2
  h_thin : Inport  Port=3
  n_thin : Inport  Port=4
  Compare To Constant : simulink/Logic and Bit Operations/Compare To Constant  relop=>=  const=Lt  OutDataTypeStr=boolean
  Constant2 : Constant  Value=Mag_legno3
  Constant3 : Constant  Value=Mag_D3
  Integrator : Integrator  ExternalReset=rising
  MATLAB Function : MATLAB Function  TreatAsAtomicUnit=on
  MATLAB Function2 : MATLAB Function  TreatAsAtomicUnit=on
  Memory : Memory
  Memory1 : Memory
  Scope{1..2,8..9} (4 alike) : Scope
  Selezione Diametro : Selector  IndexMode=Zero-based  InputPortWidth=length(Mag_D3)  IndexOptions=Index vector (port)  Indices=[1 3]  OutputSizes=1
  Selezione Tronco : Selector  IndexMode=Zero-based  InputPortWidth=length(Mag_legno3)  IndexOptions=Index vector (port)  Indices=[1 3]  OutputSizes=1
  To Workspace : ToWorkspace  VariableName=n_tronchi_3  SaveFormat=Timeseries  SampleTime=-1
  n_assi : Outport
  l_a : Outport  Port=2
  Nt : Outport  Port=3
  h : Outport  Port=4
  Dt : Outport  Port=5
  Tronco Finito : Outport  Port=6
  wires:
  MATLAB Function2/3(thickness) -> h/1
  n_thin/1 -> MATLAB Function2/4(thin_cut)
  h_thin/1 -> MATLAB Function2/3(spessore2)
  h_thick/1 -> MATLAB Function2/1(spessore)
  Compare To Constant/1 -> MATLAB Function2/2(u), Memory/1, Scope1/1
  MATLAB Function2/2(larg_asse) -> l_a/1
  Selezione Tronco/1 -> Nt/1
  MATLAB Function2/1(y) -> n_assi/1
  MATLAB Function/1(y) -> To Workspace/1, Selezione Tronco/2, Scope2/1, Selezione Diametro/2
  Constant3/1 -> Selezione Diametro/1
  Integrator/1 -> Scope8/1, Compare To Constant/1
  v1/1 -> Integrator/1
  Constant2/1 -> Selezione Tronco/1
  Memory1/1 -> MATLAB Function2/5(diametro)
  Memory/1 -> Integrator/2
  Selezione Diametro/1 -> Memory1/1, Dt/1
  MATLAB Function2/4(finito) -> Tronco Finito/1, Scope9/1, MATLAB Function/1(u)

== system SegheriaSCADA2/Linea 3/Macchina 2/Dinamica Macchina 2 ==
  n_seghe : Inport
  kc : Inport  Port=2
  h : Inport  Port=3
  Constant : Constant  Value=Tloss2
  Constant1 : Constant  Value=i_id2
  Constant4 : Constant  Value=0
  Multiply : Gain  Gain=b2/omega2
  Multiply1 : Gain  Gain=1/Kt2
  Multiply2 : Gain  Gain=1/SR2
  PID Controller : slpidlib/PID Controller  Controller=PID  Form=Parallel  TimeDomain=Continuous-time  UseExternalTs=off  SampleTime=-1  IntegratorMethod=Forward Euler  FilterMethod=Forward Euler  ControllerParametersSource=internal  P=0.1  I=0  UseKiTs=off  D=0  UseExternalDerivativeSource=off  N=100  UseFilter=on  TunerSelectOption=Transfer Function Based (PID Tuner App)  InitialConditionSource=internal  InitialConditionForIntegrator=0  InitialConditionForFilter=0  DifferentiatorICPrevScaledInput=0  ExternalReset=none  TrackingMode=off  Kt=1  LimitOutput=off  SatLimitsSource=internal  UpperSaturationLimit=1.7  LowerSaturationLimit=0  LinearizeAsGain=on  AntiWindupMode=none  Kb=1  LimitIntegrator=off  UpperIntegratorSaturationLimit=inf  LowerIntegratorSaturationLimit=-inf  POutMin=[]  POutMax=[]  IOutMin=[]  IOutMax=[]  DOutMin=[]  DOutMax=[]  NOutMin=[]  NOutMax=[]  SumOutMin=[]  SumOutMax=[]  SaturationOutMin=[]  SaturationOutMax=[]  PParamMin=[]  PParamMax=[]  IParamMin=[]  IParamMax=[]  DParamMin=[]  DParamMax=[]  NParamMin=[]  NParamMax=[]  KbParamMin=[]  KbParamMax=[]  KtParamMin=[]  KtParamMax=[]  KbOutMin=[]  KbOutMax=[]  KtOutMin=[]  KtOutMax=[]  IntegratorOutMin=[]  IntegratorOutMax=[]  FilterOutMin=[]  FilterOutMax=[]  SumI1OutMin=[]  SumI1OutMax=[]  SumI2OutMin=[]  SumI2OutMax=[]  SumI3OutMin=[]  SumI3OutMax=[]  SumI4OutMin=[]  SumI4OutMax=[]  SumDOutMin=[]  SumDOutMax=[]  DifferentiatorOutMin=[]  DifferentiatorOutMax=[]  FilterDiffOutCoefMin=[]  FilterDiffOutCoefMax=[]  ReciprocalOutMin=[]  ReciprocalOutMax=[]  SumDenOutMin=[]  SumDenOutMax=[]  SumNumOutMin=[]  SumNumOutMax=[]  DivideOutMin=[]  DivideOutMax=[]  UdiffTsProdOutMin=[]  UdiffTsProdOutMax=[]  NTsProdOutMin=[]  NTsProdOutMax=[]  UintegralTsProdOutMin=[]  UintegralTsProdOutMax=[]  UngainTsProdOutMin=[]  UngainTsProdOutMax=[]  ClampingZeroOutDataTypeStr=Inherit: Inherit via back propagation  ClampingZeroOutMin=[]  ClampingZeroOutMax=[]  FilterDenConstantOutDataTypeStr=Inherit: Inherit via back propagation  FilterDenConstantOutMin=[]  FilterDenConstantOutMax=[]  PCopyOutDataTypeStr=Inherit: Inherit via back propagation  PCopyOutMin=[]  PCopyOutMax=[]  NCopyOutDataTypeStr=Inherit: Inherit via back propagation  NCopyOutMin=[]  NCopyOutMax=[]  IntegratorContinuousStateAttributes=''  IntegratorStateMustResolveToSignalObject=off  IntegratorRTWStateStorageClass=Auto  FilterContinuousStateAttributes=''  FilterStateMustResolveToSignalObject=off  FilterRTWStateStorageClass=Auto  ParallelPVariant=InternalParameters  IdealPVariant=Disabled  IVariant=InternalParameters  DVariant=InternalParameters  IntegratorVariant=Continuous  SatVariant=Disabled  AWVariant=Passthrough  PCopyVariant=Disabled  TRVariant=Disabled  FdbkBlocksVariant=Forward  IdealPFdbkVariant=Disabled  SatFdbkVariant=Disabled  DerivativeFilterVariant=ContFilter  NVariant=InternalParameters  NCopyVariant=Disabled  FilterICVariant=InternalICsFilter  IntegratorICVariant=InternalICs  ExternalResetVariant=Disabled  TRSumVariant=Passthrough  SumFdbkVariant=Disabled  SumVariant=Sum_PID  TsampFilterVariant=InternalTs  TsampNgainVariant=Passthrough  TsampIntegralVariant=Disabled_SignalSpec  ExternalSaturationOutDataTypeStr=Inherit: Same as second input  DerivativeSourceVariant=ErrorSignal  PreIntVariant=InternalPreInt
  Product : Product  Inputs=4
  Product1 : Product
  Product2 : Product
  Scope{1..2,4..5} (4 alike) : Scope
  Sum : Sum  Inputs=+-|
  Sum1 : Sum  Inputs=++|
  Switch1 : Switch  Criteria=u2 > Threshold  SaturateOnIntegerOverflow=off  InputSameDT=off
  v1 : Outport
  tag scope: i8=global
  wires:
  [work] -> Product1/2
  Product1/1 -> Product/4, Switch1/2
  Multiply/1 -> Product1/1
  n_seghe/1 -> Product/3
  h/1 -> Product/2
  Constant/1 -> Sum1/1
  Sum1/1 -> Multiply1/1, Scope5/1
  Multiply2/1 -> Sum1/2, Scope1/1
  Sum/1 -> PID Controller/1
  Constant1/1 -> Sum/1
  Switch1/1 -> Product/1, v1/1
  kc/1 -> Multiply/1
  Multiply1/1 -> Product2/1  "iq"
  PID Controller/1 -> Scope2/1, Switch1/1
  Product/1 -> Multiply2/1, Scope4/1
  Constant4/1 -> Switch1/3
  Product2/1 -> [i8], Sum/2
  [work] -> Product2/2

== system SegheriaSCADA2/Linea 3/Macchina 3/Dinamica Macchina 2 ==
  n_seghe : Inport
  kc : Inport  Port=2
  h : Inport  Port=3
  Constant : Constant  Value=Tloss2
  Constant1 : Constant  Value=i_id2
  Constant4 : Constant  Value=0
  Multiply : Gain  Gain=b2/omega2
  Multiply1 : Gain  Gain=1/Kt2
  Multiply2 : Gain  Gain=1/SR2
  PID Controller : slpidlib/PID Controller  Controller=PID  Form=Parallel  TimeDomain=Continuous-time  UseExternalTs=off  SampleTime=-1  IntegratorMethod=Forward Euler  FilterMethod=Forward Euler  ControllerParametersSource=internal  P=0.1  I=0  UseKiTs=off  D=0  UseExternalDerivativeSource=off  N=100  UseFilter=on  TunerSelectOption=Transfer Function Based (PID Tuner App)  InitialConditionSource=internal  InitialConditionForIntegrator=0  InitialConditionForFilter=0  DifferentiatorICPrevScaledInput=0  ExternalReset=none  TrackingMode=off  Kt=1  LimitOutput=off  SatLimitsSource=internal  UpperSaturationLimit=1.7  LowerSaturationLimit=0  LinearizeAsGain=on  AntiWindupMode=none  Kb=1  LimitIntegrator=off  UpperIntegratorSaturationLimit=inf  LowerIntegratorSaturationLimit=-inf  POutMin=[]  POutMax=[]  IOutMin=[]  IOutMax=[]  DOutMin=[]  DOutMax=[]  NOutMin=[]  NOutMax=[]  SumOutMin=[]  SumOutMax=[]  SaturationOutMin=[]  SaturationOutMax=[]  PParamMin=[]  PParamMax=[]  IParamMin=[]  IParamMax=[]  DParamMin=[]  DParamMax=[]  NParamMin=[]  NParamMax=[]  KbParamMin=[]  KbParamMax=[]  KtParamMin=[]  KtParamMax=[]  KbOutMin=[]  KbOutMax=[]  KtOutMin=[]  KtOutMax=[]  IntegratorOutMin=[]  IntegratorOutMax=[]  FilterOutMin=[]  FilterOutMax=[]  SumI1OutMin=[]  SumI1OutMax=[]  SumI2OutMin=[]  SumI2OutMax=[]  SumI3OutMin=[]  SumI3OutMax=[]  SumI4OutMin=[]  SumI4OutMax=[]  SumDOutMin=[]  SumDOutMax=[]  DifferentiatorOutMin=[]  DifferentiatorOutMax=[]  FilterDiffOutCoefMin=[]  FilterDiffOutCoefMax=[]  ReciprocalOutMin=[]  ReciprocalOutMax=[]  SumDenOutMin=[]  SumDenOutMax=[]  SumNumOutMin=[]  SumNumOutMax=[]  DivideOutMin=[]  DivideOutMax=[]  UdiffTsProdOutMin=[]  UdiffTsProdOutMax=[]  NTsProdOutMin=[]  NTsProdOutMax=[]  UintegralTsProdOutMin=[]  UintegralTsProdOutMax=[]  UngainTsProdOutMin=[]  UngainTsProdOutMax=[]  ClampingZeroOutDataTypeStr=Inherit: Inherit via back propagation  ClampingZeroOutMin=[]  ClampingZeroOutMax=[]  FilterDenConstantOutDataTypeStr=Inherit: Inherit via back propagation  FilterDenConstantOutMin=[]  FilterDenConstantOutMax=[]  PCopyOutDataTypeStr=Inherit: Inherit via back propagation  PCopyOutMin=[]  PCopyOutMax=[]  NCopyOutDataTypeStr=Inherit: Inherit via back propagation  NCopyOutMin=[]  NCopyOutMax=[]  IntegratorContinuousStateAttributes=''  IntegratorStateMustResolveToSignalObject=off  IntegratorRTWStateStorageClass=Auto  FilterContinuousStateAttributes=''  FilterStateMustResolveToSignalObject=off  FilterRTWStateStorageClass=Auto  ParallelPVariant=InternalParameters  IdealPVariant=Disabled  IVariant=InternalParameters  DVariant=InternalParameters  IntegratorVariant=Continuous  SatVariant=Disabled  AWVariant=Passthrough  PCopyVariant=Disabled  TRVariant=Disabled  FdbkBlocksVariant=Forward  IdealPFdbkVariant=Disabled  SatFdbkVariant=Disabled  DerivativeFilterVariant=ContFilter  NVariant=InternalParameters  NCopyVariant=Disabled  FilterICVariant=InternalICsFilter  IntegratorICVariant=InternalICs  ExternalResetVariant=Disabled  TRSumVariant=Passthrough  SumFdbkVariant=Disabled  SumVariant=Sum_PID  TsampFilterVariant=InternalTs  TsampNgainVariant=Passthrough  TsampIntegralVariant=Disabled_SignalSpec  ExternalSaturationOutDataTypeStr=Inherit: Same as second input  DerivativeSourceVariant=ErrorSignal  PreIntVariant=InternalPreInt
  Product : Product  Inputs=4
  Product1 : Product
  Product2 : Product
  Scope{1..2,4..5} (4 alike) : Scope
  Sum : Sum  Inputs=+-|
  Sum1 : Sum  Inputs=++|
  Switch1 : Switch  Criteria=u2 > Threshold  SaturateOnIntegerOverflow=off  InputSameDT=off
  v1 : Outport
  tag scope: i9=global
  wires:
  [work] -> Product1/2
  Product1/1 -> Product/4, Switch1/2
  Multiply/1 -> Product1/1
  Constant4/1 -> Switch1/3
  Product/1 -> Scope4/1, Multiply2/1
  PID Controller/1 -> Switch1/1, Scope2/1
  Multiply1/1 -> Product2/1  "iq"
  kc/1 -> Multiply/1
  Switch1/1 -> v1/1, Product/1
  Constant1/1 -> Sum/1
  Sum/1 -> PID Controller/1
  Multiply2/1 -> Scope1/1, Sum1/2
  Sum1/1 -> Scope5/1, Multiply1/1
  Constant/1 -> Sum1/1
  h/1 -> Product/2
  n_seghe/1 -> Product/3
  Product2/1 -> [i9], Sum/2
  [work] -> Product2/2

== matlab function SegheriaSCADA2/Linea 1/MATLAB Function1 ==
  data: u input; y output
function y = fcn(u)

    persistent n_prec

    if isempty(n_prec)
        n_prec = 0;
    end

    y = u - n_prec;

    n_prec = u;

== matlab function SegheriaSCADA2/Subsystem1/MATLAB Function4 ==
  data: u input; idx output; h_index parameter
function idx = find_index(u, h_index)
%#codegen

v = h_index;

idx = -1; % valore default se non trovato

for i = 1:length(v)
    if u == v(i)
        idx = i;
        return;
    end
end

== matlab function SegheriaSCADA2/Subsystem1/MATLAB Function5 ==
  data: u input; idx output; l_index parameter
function idx = find_index(u, l_index)
%#codegen

v = l_index;

idx = -1; % valore default se non trovato

for i = 1:length(v)
    if u == v(i)
        idx = i;
        return;
    end
end

== matlab function SegheriaSCADA2/Linea 2/MATLAB Function ==
  data: u input; y output
function y = fcn(u)

    persistent n_prec

    if isempty(n_prec)
        n_prec = 0;
    end

    y = u - n_prec;


    n_prec = u;

== matlab function SegheriaSCADA2/Linea 2/MATLAB Function1 ==
  data: u input; y output
function y = fcn(u)

    persistent n_prec

    if isempty(n_prec)
        n_prec = 0;
    end

    y = u - n_prec;

    n_prec = u;

== matlab function SegheriaSCADA2/Linea 2/Macchina 1/Logica Macchina 1/MATLAB Function ==
  data: u input; y output; Mag_legno2 parameter
function y = fcn(u, Mag_legno2)
    persistent counter
    if isempty(counter)
        counter = 1;
    end

    if u == 1
        counter = counter + 1;
    end

    y = counter;
    
    if y > length(Mag_legno2)-1
        y = 0;
    end

end

== matlab function SegheriaSCADA2/Linea 2/Macchina 1/Logica Macchina 1/MATLAB Function2 ==
  settings: updateMethod=DISCRETE
  data: spessore input; u input; spessore2 input; thin_cut input; diametro input; y output; larg_asse output; thickness output; finito output
function [y, larg_asse, thickness, finito]= fcn(spessore, u, spessore2, thin_cut, diametro)
    persistent counter 

  
    max_assi = floor((diametro-thin_cut*spessore2) / spessore);
    finito = 0;
    
    if isempty(counter)
        counter = 0;
    end

    % Conto assi tagliate
    if u == 1
        counter = counter + 1;
    end

    % Quando finisco tronco segnalo e azzero counter
    if counter > max_assi + thin_cut
        finito = 1;
        counter = 0;
    end

    
    if counter == 0
        larg_asse = 0;
        thickness = 0;
    elseif counter <= thin_cut/2
        distanza_bordo = counter * spessore2;
        h = abs(diametro/2 - distanza_bordo + (spessore2/2));
        larg_asse = 2 * sqrt((diametro/2)^2-h^2);
        thickness = spessore2;
    elseif counter > max_assi + thin_cut/2
        distanza_bordo = max_assi*spessore + (counter-max_assi)*spessore2;
        h = abs(diametro/2 - distanza_bordo + (spessore2/2));
        larg_asse = 2 * sqrt((diametro/2)^2-h^2);
        thickness = spessore2;
    else
        % Calcolo larghezza delle assi
        distanza_bordo = thin_cut/2 * spessore2 + (counter-thin_cut/2) * spessore;
        h = abs(diametro/2 - distanza_bordo + (spessore/2));
        larg_asse = 2 * sqrt((diametro/2)^2-h^2);
        thickness = spessore;
    end
    

    y = counter;
